simulink model "ENV"  (R2024b)
settings: Solver=FixedStepDiscrete  StartTime=0.0  StopTime=10.0  FixedStep=0.0005  RelTol=1e-3
libraries: stm32blockslib x57, canmsglib x29, simulink x8, stm32f4xxblockslib x2
(part 5 of 5)

== matlab function ENV/CAN Rx/MATLAB Function8 ==
  data: RxBytes input uint8 size=14; Message output Bus: CAN_MESSAGE_def
function Message = DecodeCANMsg(RxBytes)
%#codegen

% rxBytes is uint8(1x14); byte 1 is the command echo (don't care)
SIDH = RxBytes(2);
SIDL = RxBytes(3);
EID8 = RxBytes(4);  %#ok — not used for standard frames
EID0 = RxBytes(5);  %#ok
DLC  = RxBytes(6);

% Assemble standard 11-bit ID
Message.ID       = uint32(bitor(uint32(bitshift(uint32(SIDH), 3)), ...
                            uint32(bitshift(uint32(SIDL), -5))));
Message.Extended = false;
Message.Remote   = false;
Message.Error    = false;
Message.Length   = double(bitand(DLC, uint8(15)));
Message.Data     = RxBytes(7:14);

== matlab function ENV/CAN Tx15/MATLAB Function ==
  settings: updateMethod=DISCRETE  sampleTime=.001
  data: WriteInstruction output; ID input uint32; CANVector output uint8; Length input uint8; Data input uint8; RTS input; RTSByte output; period input; offset input; MCPInitialized input
function [WriteInstruction, CANVector, RTSByte] = ConvertToVector(ID, Length, Data, RTS, period, offset, MCPInitialized)
%#codegen
persistent count;
if isempty(count)
    count = uint16(0);
end

if MCPInitialized
    if count == uint16(offset)
        id_u16 = uint16(ID);
        CANVector = zeros(1,13,'uint8');
        CANVector(1) = uint8(bitshift(id_u16, -3));
        CANVector(2) = uint8(bitshift(bitand(id_u16, uint16(7)), 5));
        CANVector(3) = uint8(0);
        CANVector(4) = uint8(0);
        CANVector(5) = bitand(uint8(Length), uint8(15));
        for i = 1:8
            CANVector(5+i) = uint8(Data(i));
        end
        RTSByte = uint8(RTS);
        WriteInstruction = uint8(0x02);
    else
        CANVector = zeros(1,13,'uint8');
        RTSByte = uint8(RTS);
        WriteInstruction = uint8(0x03);
    end

    count = count + uint16(1);
    if count >= uint16(period)
        count = uint16(0);
    end
else
    CANVector = zeros(1,13,'uint8');
    RTSByte = uint8(0x03);
    WriteInstruction = uint8(0x03);
    % don't increment count while MCP not ready
end
